simulink model "QuadcopterSimModel_ArduCopter_SITL"  (R2018b)
settings: Solver=ode23  StartTime=0.0  StopTime=1000  FixedStep=sample_time  RelTol=1e-4  EnableMultiTasking=on
undefined symbols (not defined in the file): alt_ground, atmosphere, envir, g, pos_ref, wind
libraries: ardupilot_sitl_lib x3, unit_conversions_lib x3, flightgear_visualization_lib x2, atmosphere_lib x1, quadcopter_lib x1, sensors_lib x1, simulink x1, axes_transformation_lib x1
settings Model: SimulationMode=accelerator  EnablePacing=on  Creator=Yannic  LastModifiedBy=yannic
settings SolverCC: ZeroCrossControl=DisableAll
settings DataIOCC: LimitDataPoints=on  ReturnWorkspaceOutputs=on
settings OptimizationCC: LifeSpan=inf
settings DebuggingCC: ReadBeforeWriteMsg=DisableAll  WriteAfterWriteMsg=DisableAll  WriteAfterReadMsg=DisableAll  MultiTaskDSMMsg=none  AllowSymbolicDim=off  SFUnexpectedBacktrackingDiag=warning  SFNoUnconditionalDefaultTransitionDiag=warning  SFExecutionAtInitializationDiag=none
settings ModelReferenceCC: UpdateModelReferenceTargets=IfOutOfDate  PropagateSignalLabelsOutOfModel=off
settings SFSimCC: SFSimEcho=off  SimUseLocalCustomCode=off
settings RTWCC: RTWUseLocalCustomCode=off
settings CodeAppCC: StateflowObjectComments=on
settings GRTTargetCC: TargetLangStandard=C89/C90 (ANSI)
settings ConfigComp: CovMetricSettings=dw  CovSaveCumulativeToWorkspaceVar=on  CovSaveSingleToWorkspaceVar=on  CovExternalEMLEnable=off

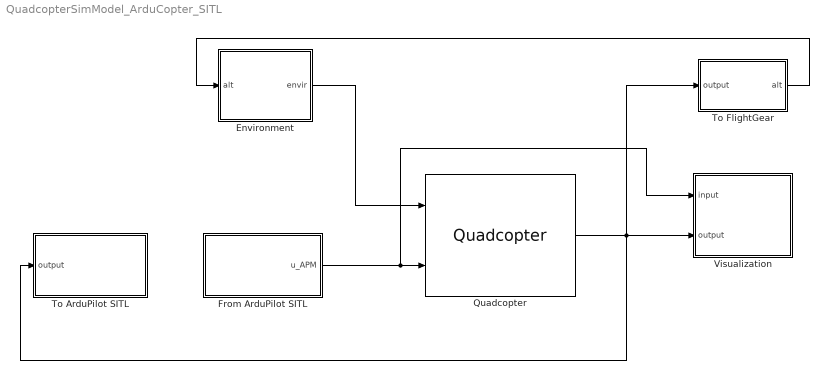
== system QuadcopterSimModel_ArduCopter_SITL ==
  Environment : Subsystem
  From ArduPilot SITL : Subsystem
  Quadcopter : quadcopter_lib/Quadcopter  copter_=copter  IC_=IC  grnd_=grnd
      settings: SourceProductName=LADAC
  To ArduPilot SITL : Subsystem
  To FlightGear : Subsystem
  Visualization : Subsystem
  wires:
  Environment/1(envir) -> Quadcopter/1
  Quadcopter/1 -> To FlightGear/1(output), Visualization/2(output), To ArduPilot SITL/1(output)
  To FlightGear/1(alt) -> Environment/1(alt)
  From ArduPilot SITL/1(u_APM) -> Quadcopter/2, Visualization/1(input)

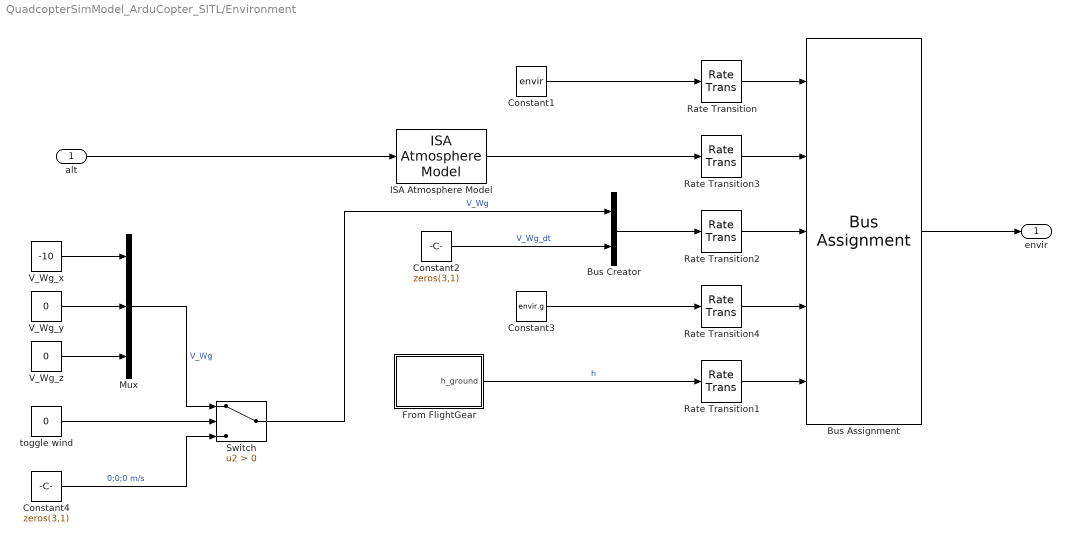
== system QuadcopterSimModel_ArduCopter_SITL/Environment ==
  alt : Inport
  Bus Assignment : BusAssignment  AssignedSignals=atmosphere,wind,g,alt_ground
  Bus Creator : BusCreator  Inputs=2
  Constant1 : Constant  Value=envir  OutDataTypeStr=Bus: envirBus
  Constant2 : Constant  Value=zeros(3,1)
  Constant3 : Constant  Value=envir.g
  Constant4 : Constant  Value=zeros(3,1)
  From FlightGear : Subsystem
  ISA Atmosphere Model : atmosphere_lib/ISA Atmosphere Model
      settings: SourceProductName=LADAC
  Mux : Mux  Inputs=3
  Rate Transition{,1..4} (5 alike) : RateTransition
  Switch : Switch  Criteria=u2 > Threshold
  V_Wg_x : Constant  Value=-10
  V_Wg_y : Constant  Value=0
  V_Wg_z : Constant  Value=0
  toggle wind : Constant  Value=0
  envir : Outport
  wires:
  From FlightGear/1(h_ground) -> Rate Transition1/1  "h"
  Rate Transition2/1 -> Bus Assignment/3
  Rate Transition3/1 -> Bus Assignment/2
  Bus Assignment/1 -> envir/1
  Rate Transition/1 -> Bus Assignment/1
  ISA Atmosphere Model/1 -> Rate Transition3/1
  Switch/1 -> Bus Creator/1  "V_Wg"
  Rate Transition1/1 -> Bus Assignment/5
  Constant1/1 -> Rate Transition/1
  alt/1 -> ISA Atmosphere Model/1
  Bus Creator/1 -> Rate Transition2/1
  Constant2/1 -> Bus Creator/2  "V_Wg_dt"
  Rate Transition4/1 -> Bus Assignment/4
  Constant3/1 -> Rate Transition4/1
  V_Wg_x/1 -> Mux/1
  V_Wg_y/1 -> Mux/2
  V_Wg_z/1 -> Mux/3
  Mux/1 -> Switch/1  "V_Wg"
  Constant4/1 -> Switch/3  "0;0;0 m/s"
  toggle wind/1 -> Switch/2

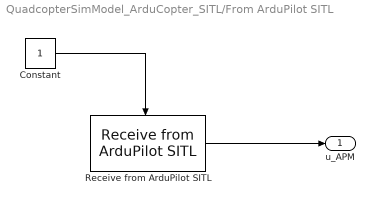
== system QuadcopterSimModel_ArduCopter_SITL/From ArduPilot SITL ==
  Constant : Constant
  Receive from ArduPilot SITL : ardupilot_sitl_lib/Receive from ArduPilot SITL  idx=[3,1,4,2]  IP='127.0.0.1'  Port=9002  sample_time=SITL.sample_time  blocking_time=1
      settings: SourceProductName=LADAC
  u_APM : Outport
  wires:
  Receive from ArduPilot SITL/1 -> u_APM/1
  Constant/1 -> Receive from ArduPilot SITL/Enable

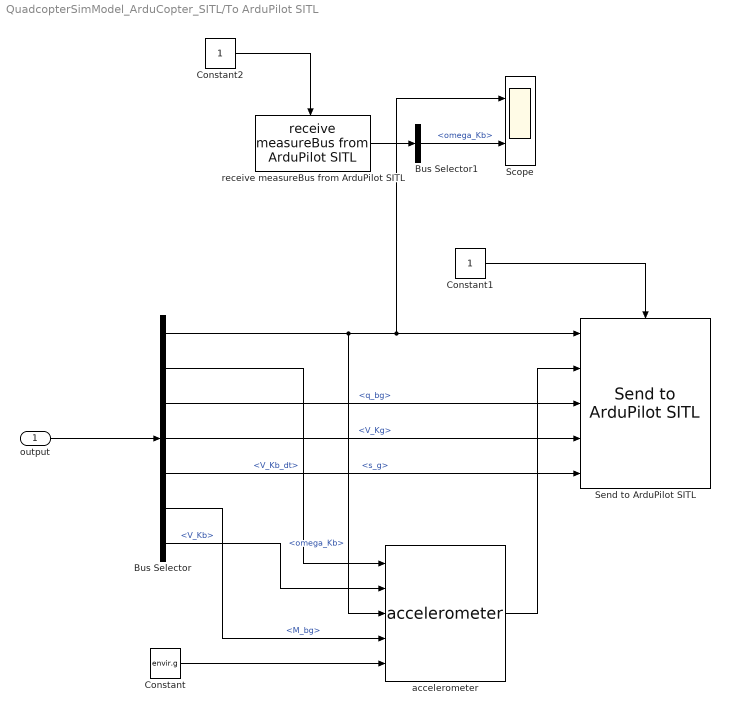
== system QuadcopterSimModel_ArduCopter_SITL/To ArduPilot SITL ==
  output : Inport
  Bus Selector : BusSelector  OutputSignals=rigidBodyBus.omega_Kb,rigidBodyBus.V_Kb_dt,rigidBodyBus.q_bg,rigidBodyBus.V_Kg,rigidBodyBus.s_g,rigidBodyBus.M_bg,rigidBodyBus.V_Kb
  Bus Selector1 : BusSelector  OutputSignals=omega_Kb
  Constant : Constant  Value=envir.g
  Constant1 : Constant
  Constant2 : Constant
  Scope : Scope  NumInputPorts=2
  Send to ArduPilot SITL : ardupilot_sitl_lib/Send to ArduPilot SITL  IP='127.0.0.1'  Port=9003  sample_time=SITL.sample_time
      settings: SourceProductName=LADAC
  accelerometer : sensors_lib/accelerometer  SystemSampleTime=-1
      settings: SourceProductName=LADAC
  receive measureBus from ArduPilot SITL : ardupilot_sitl_lib/receive measureBus  from ArduPilot SITL  IP='127.0.0.1'  Port=9004  sample_time=1/400  blocking_time=0.001
      settings: SourceProductName=LADAC
  wires:
  Bus Selector/4 -> Send to ArduPilot SITL/4  "<V_Kg>"
  Bus Selector/3 -> Send to ArduPilot SITL/3  "<q_bg>"
  Bus Selector/2 -> accelerometer/1  "<V_Kb_dt>"
  Bus Selector/1 -> accelerometer/3, Scope/1, Send to ArduPilot SITL/1  "<omega_Kb>"
  Bus Selector/5 -> Send to ArduPilot SITL/5  "<s_g>"
  output/1 -> Bus Selector/1
  Bus Selector/6 -> accelerometer/4  "<M_bg>"
  Constant/1 -> accelerometer/5
  accelerometer/1 -> Send to ArduPilot SITL/2
  Constant1/1 -> Send to ArduPilot SITL/Enable
  Bus Selector/7 -> accelerometer/2  "<V_Kb>"
  receive measureBus from ArduPilot SITL/1 -> Bus Selector1/1
  Bus Selector1/1 -> Scope/2  "<omega_Kb>"
  Constant2/1 -> receive measureBus from ArduPilot SITL/Enable

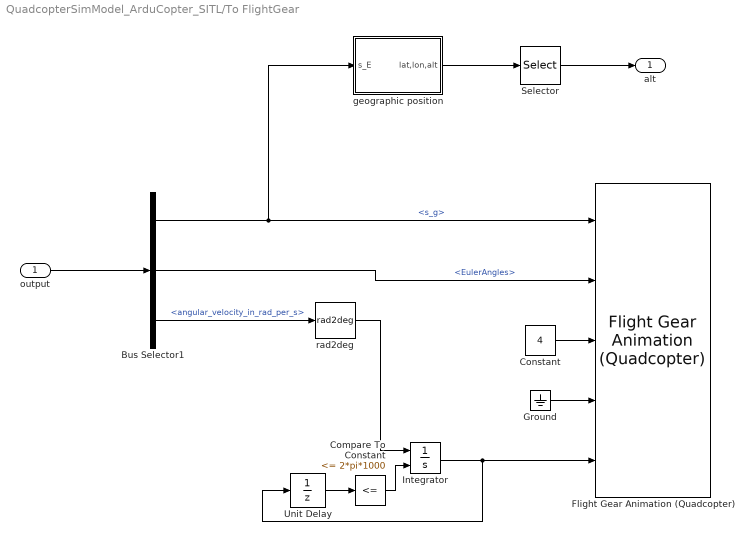
== system QuadcopterSimModel_ArduCopter_SITL/To FlightGear ==
  output : Inport
  Bus Selector1 : BusSelector  OutputSignals=rigidBodyBus.s_g,rigidBodyBus.EulerAngles,motorBus.angular_velocity_in_rad_per_s
  Compare To Constant : simulink/Logic and Bit Operations/Compare To Constant  relop=<=  const=2*pi*1000  OutDataTypeStr=boolean
  Constant : Constant  Value=4
  Flight Gear Animation (Quadcopter) : flightgear_visualization_lib/Flight Gear Animation (Quadcopter)  inital_lat=pos_ref.lat  inital_long=pos_ref.lon  inital_height=pos_ref.alt  remoteURL=fg.remoteURL  remotePort=fg.remotePort
      settings: SourceProductName=LADAC
  Ground : Ground
  Integrator : Integrator  ExternalReset=rising
  Selector : Selector  InputPortWidth=3  IndexOptions=Index vector (dialog)  Indices=3  OutputSizes=1
  Unit Delay : UnitDelay  SampleTime=-1
  geographic position : Subsystem
  rad2deg : unit_conversions_lib/rad2deg
      settings: SourceProductName=LADAC
  alt : Outport
  wires:
  output/1 -> Bus Selector1/1
  geographic position/1(lat,lon,alt) -> Selector/1
  Selector/1 -> alt/1
  Constant/1 -> Flight Gear Animation (Quadcopter)/3
  Ground/1 -> Flight Gear Animation (Quadcopter)/4
  Integrator/1 -> Unit Delay/1, Flight Gear Animation (Quadcopter)/5
  Unit Delay/1 -> Compare To Constant/1
  Compare To Constant/1 -> Integrator/2
  rad2deg/1 -> Integrator/1
  Bus Selector1/1 -> geographic position/1(s_E), Flight Gear Animation (Quadcopter)/1  "<s_g>"
  Bus Selector1/3 -> rad2deg/1  "<angular_velocity_in_rad_per_s>"
  Bus Selector1/2 -> Flight Gear Animation (Quadcopter)/2  "<EulerAngles>"

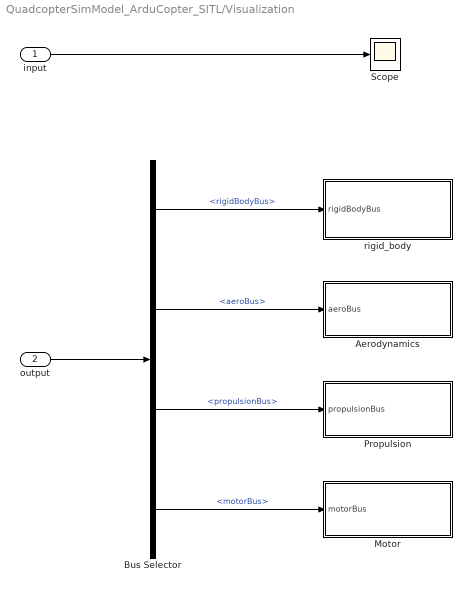
== system QuadcopterSimModel_ArduCopter_SITL/Visualization ==
  input : Inport
  output : Inport  Port=2
  Aerodynamics : Subsystem
  Bus Selector : BusSelector  OutputSignals=rigidBodyBus,aeroBus,propulsionBus,motorBus
  Motor : Subsystem
  Propulsion : Subsystem
  Scope : Scope
  rigid_body : Subsystem
  wires:
  output/1 -> Bus Selector/1
  Bus Selector/1 -> rigid_body/1(rigidBodyBus)  "<rigidBodyBus>"
  Bus Selector/2 -> Aerodynamics/1(aeroBus)  "<aeroBus>"
  Bus Selector/3 -> Propulsion/1(propulsionBus)  "<propulsionBus>"
  Bus Selector/4 -> Motor/1(motorBus)  "<motorBus>"
  input/1 -> Scope/1

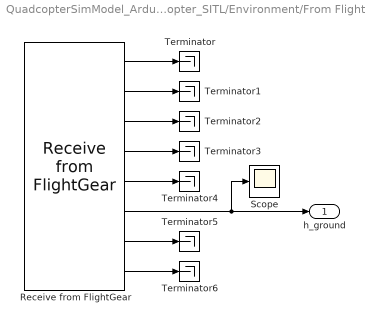
== system QuadcopterSimModel_ArduCopter_SITL/Environment/From FlightGear ==
  Receive from FlightGear : flightgear_visualization_lib/Receive from FlightGear  ip_address='127.0.0.1'  ip_port=5503  sample_time=1/30  blocking_time=0  is_aerocntrl=off  is_engine=off  is_fuel=off  is_land=off  is_avionics=off  is_envir=on
      settings: SourceProductName=LADAC
  Scope : Scope
  Terminator{,1..6} (7 alike) : Terminator
  h_ground : Outport
  wires:
  Receive from FlightGear/4 -> Terminator3/1
  Receive from FlightGear/5 -> Terminator4/1
  Receive from FlightGear/2 -> Terminator1/1
  Receive from FlightGear/7 -> Terminator5/1
  Receive from FlightGear/1 -> Terminator/1
  Receive from FlightGear/3 -> Terminator2/1
  Receive from FlightGear/8 -> Terminator6/1
  Receive from FlightGear/6 -> Scope/1, h_ground/1

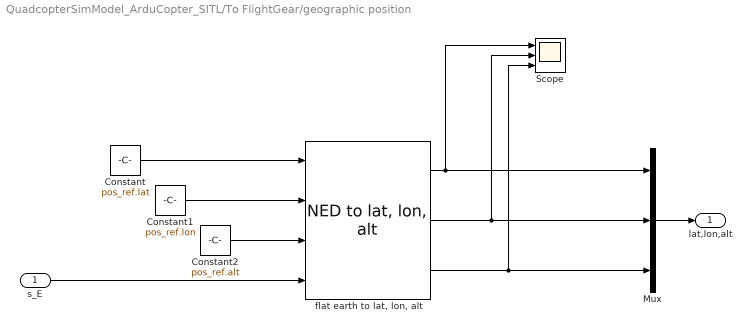
== system QuadcopterSimModel_ArduCopter_SITL/To FlightGear/geographic position ==
  s_E : Inport
  Constant : Constant  Value=pos_ref.lat
  Constant1 : Constant  Value=pos_ref.lon
  Constant2 : Constant  Value=pos_ref.alt
  Mux : Mux  Inputs=3
  Scope : Scope  NumInputPorts=3
  "flat earth to lat, lon, alt" : axes_transformation_lib/NED to lat, lon, alt  SystemSampleTime=-1
      settings: SourceProductName=LADAC
  lat,lon,alt : Outport
  wires:
  Constant2/1 -> "flat earth to lat, lon, alt"/3
  Constant1/1 -> "flat earth to lat, lon, alt"/2
  "flat earth to lat, lon, alt"/3 -> Scope/3, Mux/3
  Constant/1 -> "flat earth to lat, lon, alt"/1
  Mux/1 -> lat,lon,alt/1
  s_E/1 -> "flat earth to lat, lon, alt"/4
  "flat earth to lat, lon, alt"/2 -> Mux/2, Scope/2
  "flat earth to lat, lon, alt"/1 -> Mux/1, Scope/1

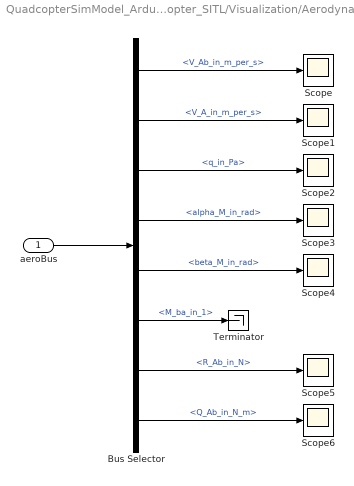
== system QuadcopterSimModel_ArduCopter_SITL/Visualization/Aerodynamics ==
  aeroBus : Inport
  Bus Selector : BusSelector  OutputSignals=V_Ab_in_m_per_s,V_A_in_m_per_s,q_in_Pa,angles.alpha_M_in_rad,angles.beta_M_in_rad,M_ba_in_1,R_Ab_in_N,Q_Ab_in_N_m
  Scope{,1..6} (7 alike) : Scope
  Terminator : Terminator
  wires:
  aeroBus/1 -> Bus Selector/1
  Bus Selector/1 -> Scope/1  "<V_Ab_in_m_per_s>"
  Bus Selector/2 -> Scope1/1  "<V_A_in_m_per_s>"
  Bus Selector/3 -> Scope2/1  "<q_in_Pa>"
  Bus Selector/4 -> Scope3/1  "<alpha_M_in_rad>"
  Bus Selector/5 -> Scope4/1  "<beta_M_in_rad>"
  Bus Selector/6 -> Terminator/1  "<M_ba_in_1>"
  Bus Selector/7 -> Scope5/1  "<R_Ab_in_N>"
  Bus Selector/8 -> Scope6/1  "<Q_Ab_in_N_m>"

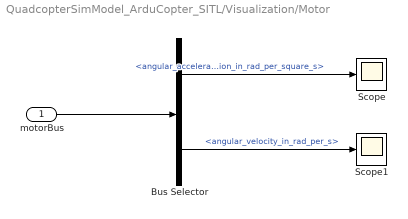
== system QuadcopterSimModel_ArduCopter_SITL/Visualization/Motor ==
  motorBus : Inport
  Bus Selector : BusSelector  OutputSignals=angular_acceleration_in_rad_per_square_s,angular_velocity_in_rad_per_s
  Scope : Scope
  Scope1 : Scope
  wires:
  Bus Selector/1 -> Scope/1  "<angular_acceleration_in_rad_per_square_s>"
  motorBus/1 -> Bus Selector/1
  Bus Selector/2 -> Scope1/1  "<angular_velocity_in_rad_per_s>"

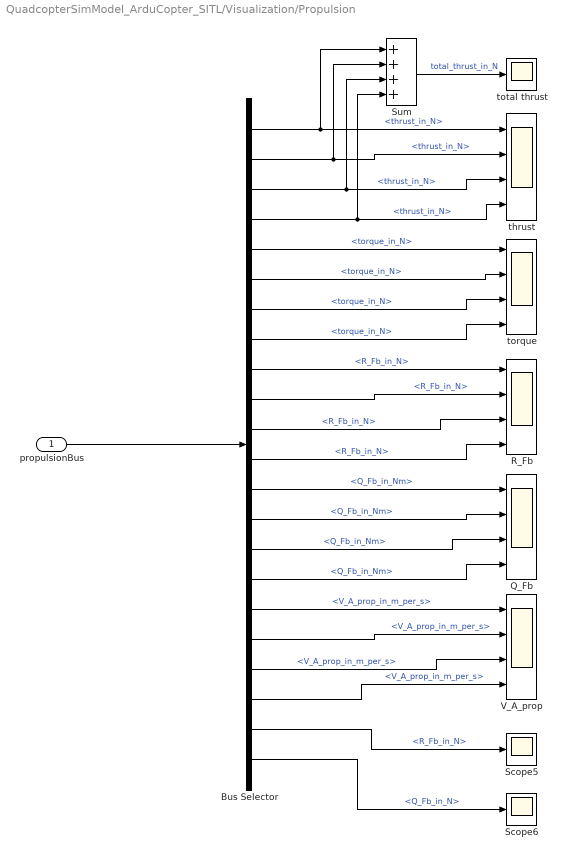
== system QuadcopterSimModel_ArduCopter_SITL/Visualization/Propulsion ==
  propulsionBus : Inport
  Bus Selector : BusSelector  OutputSignals=propeller_1.thrust_in_N,propeller_2.thrust_in_N,propeller_3.thrust_in_N,propeller_4.thrust_in_N,propeller_1.torque_in_N,propeller_2.torque_in_N,propeller_3.torque_in_N,propeller_4.torque_in_N,propeller_1.R_Fb_in_N,propeller_2.R_Fb_in_N,propeller_3.R_Fb_in_N,propeller_4.R_Fb_in_N,propeller_1.Q_Fb_in_Nm,propeller_2.Q_Fb_in_Nm,propeller_3.Q_Fb_in_Nm,propeller_4.Q_Fb_in_Nm,propeller_1.V_A_prop_in_m_per_s,propeller_2.V_A_prop_in_m_per_s,propeller_3.V_A_prop_in_m_per_s,propeller_4.V_A_prop_in_m_per_s,R_Fb_in_N,Q_Fb_in_N
  Q_Fb : Scope  NumInputPorts=4
  R_Fb : Scope  NumInputPorts=4
  Scope5 : Scope
  Scope6 : Scope
  Sum : Sum  Inputs=4
  V_A_prop : Scope  NumInputPorts=4
  thrust : Scope  NumInputPorts=4
  torque : Scope  NumInputPorts=4
  total thrust : Scope
  wires:
  propulsionBus/1 -> Bus Selector/1
  Bus Selector/1 -> Sum/1, thrust/1  "<thrust_in_N>"
  Bus Selector/2 -> Sum/2, thrust/2  "<thrust_in_N>"
  Bus Selector/3 -> Sum/3, thrust/3  "<thrust_in_N>"
  Bus Selector/4 -> Sum/4, thrust/4  "<thrust_in_N>"
  Bus Selector/5 -> torque/1  "<torque_in_N>"
  Bus Selector/6 -> torque/2  "<torque_in_N>"
  Bus Selector/7 -> torque/3  "<torque_in_N>"
  Bus Selector/8 -> torque/4  "<torque_in_N>"
  Bus Selector/9 -> R_Fb/1  "<R_Fb_in_N>"
  Bus Selector/10 -> R_Fb/2  "<R_Fb_in_N>"
  Bus Selector/11 -> R_Fb/3  "<R_Fb_in_N>"
  Bus Selector/12 -> R_Fb/4  "<R_Fb_in_N>"
  Bus Selector/13 -> Q_Fb/1  "<Q_Fb_in_Nm>"
  Bus Selector/14 -> Q_Fb/2  "<Q_Fb_in_Nm>"
  Bus Selector/15 -> Q_Fb/3  "<Q_Fb_in_Nm>"
  Bus Selector/16 -> Q_Fb/4  "<Q_Fb_in_Nm>"
  Bus Selector/17 -> V_A_prop/1  "<V_A_prop_in_m_per_s>"
  Bus Selector/18 -> V_A_prop/2  "<V_A_prop_in_m_per_s>"
  Bus Selector/19 -> V_A_prop/3  "<V_A_prop_in_m_per_s>"
  Bus Selector/20 -> V_A_prop/4  "<V_A_prop_in_m_per_s>"
  Bus Selector/21 -> Scope5/1  "<R_Fb_in_N>"
  Bus Selector/22 -> Scope6/1  "<Q_Fb_in_N>"
  Sum/1 -> total thrust/1  "total_thrust_in_N"

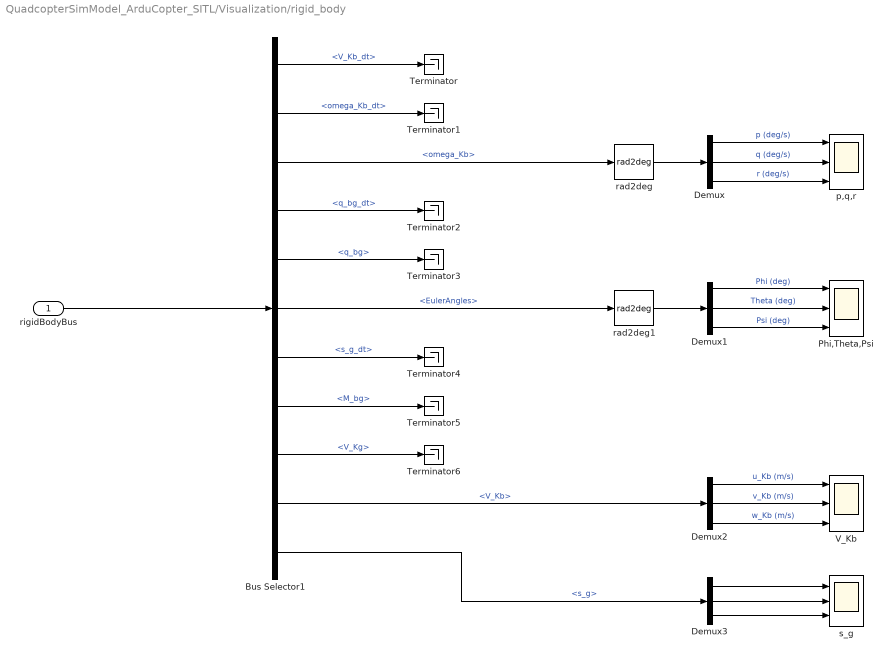
== system QuadcopterSimModel_ArduCopter_SITL/Visualization/rigid_body ==
  rigidBodyBus : Inport
  Bus Selector1 : BusSelector  OutputSignals=V_Kb_dt,omega_Kb_dt,omega_Kb,q_bg_dt,q_bg,EulerAngles,s_g_dt,M_bg,V_Kg,V_Kb,s_g
  Demux{,1..3} (4 alike) : Demux  Outputs=3
  Phi,Theta,Psi : Scope  NumInputPorts=3
  Terminator{,1..6} (7 alike) : Terminator
  V_Kb : Scope  NumInputPorts=3
  p,q,r : Scope  NumInputPorts=3
  rad2deg : unit_conversions_lib/rad2deg
      settings: SourceProductName=LADAC
  rad2deg1 : unit_conversions_lib/rad2deg
      settings: SourceProductName=LADAC
  s_g : Scope  NumInputPorts=3
  wires:
  Demux/1 -> p,q,r/1  "p (deg/s)"
  Demux1/2 -> Phi,Theta,Psi/2  "Theta (deg)"
  rad2deg/1 -> Demux/1
  Demux1/1 -> Phi,Theta,Psi/1  "Phi (deg)"
  Demux1/3 -> Phi,Theta,Psi/3  "Psi (deg)"
  Demux2/3 -> V_Kb/3  "w_Kb (m/s)"
  Bus Selector1/7 -> Terminator4/1  "<s_g_dt>"
  Bus Selector1/6 -> rad2deg1/1  "<EulerAngles>"
  Bus Selector1/3 -> rad2deg/1  "<omega_Kb>"
  Demux/3 -> p,q,r/3  "r (deg/s)"
  Bus Selector1/1 -> Terminator/1  "<V_Kb_dt>"
  Demux2/2 -> V_Kb/2  "v_Kb (m/s)"
  Demux/2 -> p,q,r/2  "q (deg/s)"
  rad2deg1/1 -> Demux1/1
  Bus Selector1/5 -> Terminator3/1  "<q_bg>"
  Demux2/1 -> V_Kb/1  "u_Kb (m/s)"
  Bus Selector1/10 -> Demux2/1  "<V_Kb>"
  rigidBodyBus/1 -> Bus Selector1/1
  Bus Selector1/8 -> Terminator5/1  "<M_bg>"
  Bus Selector1/4 -> Terminator2/1  "<q_bg_dt>"
  Bus Selector1/2 -> Terminator1/1  "<omega_Kb_dt>"
  Bus Selector1/9 -> Terminator6/1  "<V_Kg>"
  Bus Selector1/11 -> Demux3/1  "<s_g>"
  Demux3/1 -> s_g/1
  Demux3/2 -> s_g/2
  Demux3/3 -> s_g/3
